simulink model "new_control"  (R2024b)
settings: Solver=FixedStepAuto  StartTime=0.0  StopTime=inf  FixedStep=0.01  RelTol=1e-3  EnableMultiTasking=on
undefined symbols (not defined in the file or in its folder): Discrete, qbreak, Time
libraries: simulink x70, arduinolib x30, dspswit3 x13, arduinosensorlib x2, ctrlSharedLib x2
(part 1 of 4)

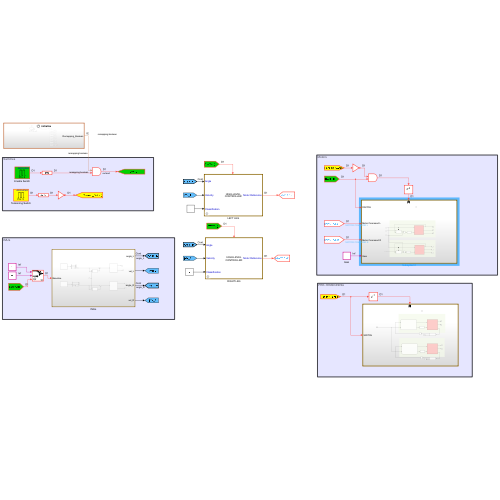
[thumbnail: Simulink's stored preview of the top-level diagram]
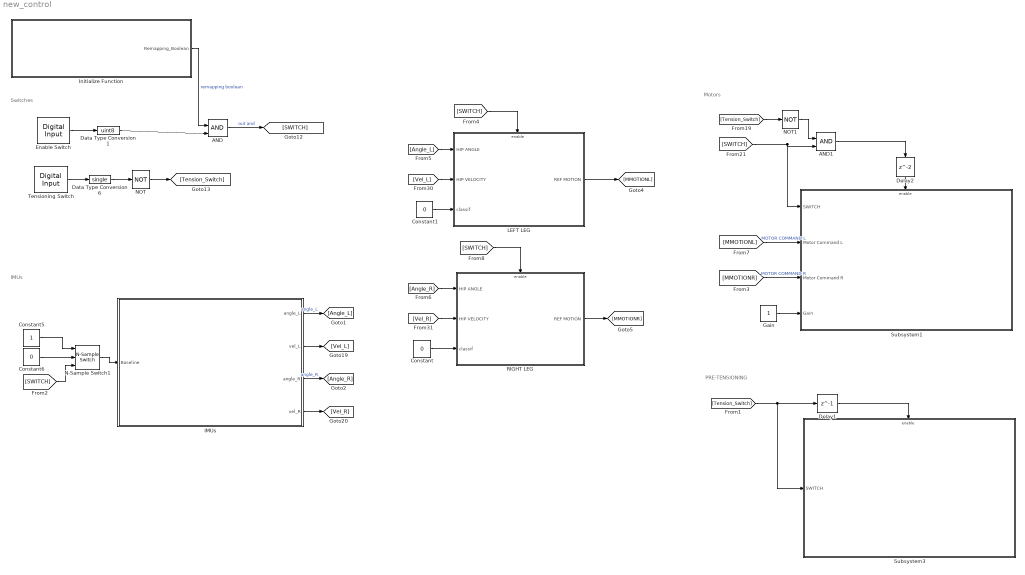
== system new_control ==
  note: Motors
  note: PRE-TENSIONING
  note: IMUs
  note: Switches
  AND : Logic  IconShape=distinctive  AllPortsSameDT=off  OutDataTypeStr=boolean
  AND1 : Logic  IconShape=distinctive  AllPortsSameDT=off  OutDataTypeStr=boolean
  Constant : Constant  Value=0
  Constant1 : Constant  Value=0
  Constant5 : Constant
  Constant6 : Constant  Value=0
  Data Type Conversion1 : DataTypeConversion  OutDataTypeStr=uint8  SaturateOnIntegerOverflow=off  RndMeth=Floor
  Data Type Conversion6 : DataTypeConversion  OutDataTypeStr=single  SaturateOnIntegerOverflow=off  RndMeth=Floor
  Delay1 : Delay  DelayLength=1
  Delay2 : Delay
  Enable Switch : arduinolib/Digital Input  pinNumber=6  mode=Default  Direction=input  SampleTime=0.01  blockPlatform=arduino
  Gain : Constant
  IMUs : Subsystem
  Initialize Function : Subsystem  TreatAsAtomicUnit=on
  LEFT LEG : Subsystem  mask{AMPL=-6.5, LAG=0, SIG_POWER=50}
      mask prompts: AMPL "Motor position desidered amplitude (rad)"; LAG "Lag compensation (rad)"; SIG_POWER "Sigmoid Power"
  N-Sample Switch1 : dspswit3/N-Sample Switch  N=10  reset=on  TriggerType=Rising edge  Ts=0.01
  NOT : Logic  Operator=NOT  IconShape=distinctive  AllPortsSameDT=off  OutDataTypeStr=boolean
  NOT1 : Logic  Operator=NOT  IconShape=distinctive  AllPortsSameDT=off  OutDataTypeStr=boolean
  RIGHT LEG : Subsystem  mask{AMPL=6.5, LAG=0, SIG_POWER=50}
      mask prompts: AMPL "Motor position desidered amplitude (rad)"; LAG "Lag compensation (rad)"; SIG_POWER "Sigmoid Power"
  Subsystem1 : Subsystem
  Subsystem3 : Subsystem
  Tensioning Switch : arduinolib/Digital Input  pinNumber=5  mode=Input Pullup  Direction=input  SampleTime=0.01  blockPlatform=arduino
  wires:
  LEFT LEG/1(REF MOTION) -> [MMOTIONL]
  Gain/1 -> Subsystem1/4(Gain)
  Delay2/1 -> Subsystem1/Enable
  NOT1/1 -> AND1/1
  AND1/1 -> Delay2/1
  [SWITCH] -> AND1/2, Subsystem1/1(SWITCH)
  [Tension_Switch] -> NOT1/1
  Delay1/1 -> Subsystem3/Enable
  [Tension_Switch] -> Subsystem3/1(SWITCH), Delay1/1
  IMUs/1(angle_L) -> [Angle_L]  "angle_L"
  N-Sample Switch1/1 -> IMUs/1(Baseline)
  Constant6/1 -> N-Sample Switch1/2
  Constant5/1 -> N-Sample Switch1/1
  IMUs/3(angle_R) -> [Angle_R]  "angle_R"
  [SWITCH] -> N-Sample Switch1/3
  [SWITCH] -> LEFT LEG/Enable
  [Angle_L] -> LEFT LEG/1(HIP ANGLE)
  Tensioning Switch/1 -> Data Type Conversion6/1
  Data Type Conversion1/1 -> AND/2
  NOT/1 -> [Tension_Switch]
  Initialize Function/1(Remapping_Boolean) -> AND/1  "remapping boolean"
  Data Type Conversion6/1 -> NOT/1
  AND/1 -> [SWITCH]  "out and"
  Enable Switch/1 -> Data Type Conversion1/1
  [Angle_R] -> RIGHT LEG/1(HIP ANGLE)
  [MMOTIONL] -> Subsystem1/2(Motor Command L)  "MOTOR COMMAND L"
  [MMOTIONR] -> Subsystem1/3(Motor Command R)  "MOTOR COMMAND R"
  RIGHT LEG/1(REF MOTION) -> [MMOTIONR]
  [SWITCH] -> RIGHT LEG/Enable
  Constant1/1 -> LEFT LEG/3(classif)
  Constant/1 -> RIGHT LEG/3(classif)
  IMUs/2(vel_L) -> [Vel_L]
  IMUs/4(vel_R) -> [Vel_R]
  [Vel_L] -> LEFT LEG/2(HIP VELOCITY)
  [Vel_R] -> RIGHT LEG/2(HIP VELOCITY)

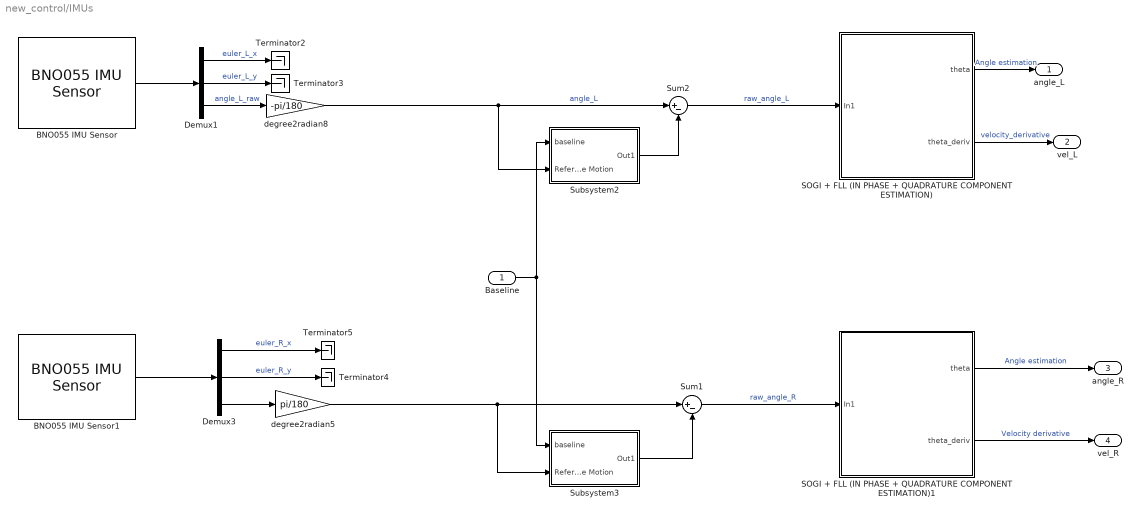
== system new_control/IMUs ==
  Baseline : Inport
  BNO055 IMU Sensor : arduinosensorlib/BNO055 IMU Sensor  I2CModule=0  SlaveAddress=0x28  OperationMode=Fusion  Accel=off  AngularRate=off  MagField=off  EulerAngles=on  Quat=off  LinearAccel=off  GravityVector=off  Status=off  Timestamp=off  AccelRange=4G  AccelBW=62.5 Hz  GyroRange=2000 dps  GyroBW=32 Hz  MagODR=10 Hz  spf=1  SampleTime=-1  blockPlatform=ARDUINO  QueueSizeFactor=1
  BNO055 IMU Sensor1 : arduinosensorlib/BNO055 IMU Sensor  I2CModule=0  SlaveAddress=0x29  OperationMode=Fusion  Accel=off  AngularRate=off  MagField=off  EulerAngles=on  Quat=off  LinearAccel=off  GravityVector=off  Status=off  Timestamp=off  AccelRange=4G  AccelBW=62.5 Hz  GyroRange=2000 dps  GyroBW=32 Hz  MagODR=10 Hz  spf=1  SampleTime=-1  blockPlatform=ARDUINO  QueueSizeFactor=1
  Demux1 : Demux  Outputs=3
  Demux3 : Demux  Outputs=3
  SOGI + FLL (IN PHASE + QUADRATURE COMPONENT ESTIMATION) : Subsystem  mask{Tsamp=0.01, fmin=0.2, fmax=4.0, ksogi=1, kfll=1.0, Elo=1e-4, Ehi=1e-2}
      mask prompts: Tsamp "Sampling time (s)"; fmin "Minimum movement frequency (Hz)"; fmax "Maximum movement frequency (Hz)"; ksogi "SOGI amplitude adaptation gain"; kfll "FLL frequency adaptation gain"; Elo "Low energy threshold"; Ehi "High energy threshold"
  SOGI + FLL (IN PHASE + QUADRATURE COMPONENT ESTIMATION)1 : Subsystem  mask{Tsamp=0.01, fmin=0.2, fmax=4.0, ksogi=1, kfll=1.0, Elo=1e-4, Ehi=1e-2}
      mask prompts: Tsamp "Sampling time (s)"; fmin "Minimum movement frequency (Hz)"; fmax "Maximum movement frequency (Hz)"; ksogi "SOGI amplitude adaptation gain"; kfll "FLL frequency adaptation gain"; Elo "Low energy threshold"; Ehi "High energy threshold"
  Subsystem2 : Subsystem
  Subsystem3 : Subsystem
  Sum1 : Sum  Inputs=|+-
  Sum2 : Sum  Inputs=|+-
  Terminator{2..5} (4 alike) : Terminator
  degree2radian5 : Gain  Gain=pi/180
  degree2radian8 : Gain  Gain=-pi/180
  angle_L : Outport
  vel_L : Outport  Port=2
  angle_R : Outport  Port=3
  vel_R : Outport  Port=4
  wires:
  BNO055 IMU Sensor/1 -> Demux1/1
  BNO055 IMU Sensor1/1 -> Demux3/1
  Demux1/1 -> Terminator2/1  "euler_L_x"
  Demux1/3 -> degree2radian8/1  "angle_L_raw"
  Demux1/2 -> Terminator3/1  "euler_L_y"
  Demux3/1 -> Terminator5/1  "euler_R_x"
  Demux3/2 -> Terminator4/1  "euler_R_y"
  Demux3/3 -> degree2radian5/1
  Sum1/1 -> SOGI + FLL (IN PHASE + QUADRATURE COMPONENT ESTIMATION)1/1(In1)  "raw_angle_R"
  Baseline/1 -> Subsystem2/1(baseline), Subsystem3/1(baseline)
  Subsystem2/1(Out1) -> Sum2/2
  degree2radian5/1 -> Subsystem3/2(Reference Motion), Sum1/1
  Subsystem3/1(Out1) -> Sum1/2
  degree2radian8/1 -> Subsystem2/2(Reference Motion), Sum2/1  "angle_L"
  Sum2/1 -> SOGI + FLL (IN PHASE + QUADRATURE COMPONENT ESTIMATION)/1(In1)  "raw_angle_L"
  SOGI + FLL (IN PHASE + QUADRATURE COMPONENT ESTIMATION)/1(theta) -> angle_L/1  "Angle estimation"
  SOGI + FLL (IN PHASE + QUADRATURE COMPONENT ESTIMATION)1/1(theta) -> angle_R/1  "Angle estimation"
  SOGI + FLL (IN PHASE + QUADRATURE COMPONENT ESTIMATION)1/2(theta_deriv) -> vel_R/1  "Velocity derivative"
  SOGI + FLL (IN PHASE + QUADRATURE COMPONENT ESTIMATION)/2(theta_deriv) -> vel_L/1  "velocity_derivative"

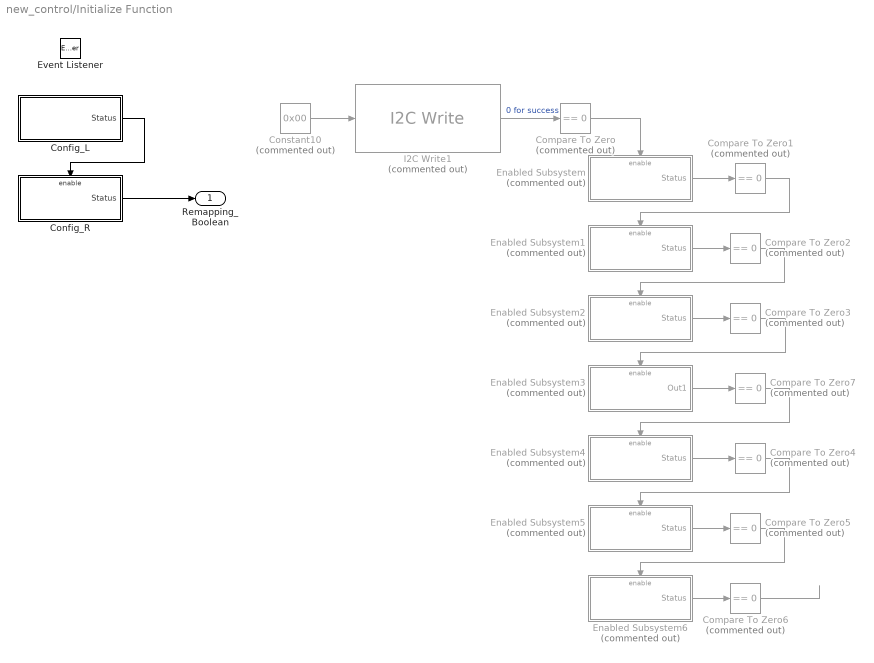
== system new_control/Initialize Function ==
  Compare To Zero{,1..7} (8 alike) : simulink/Logic and Bit Operations/Compare To Zero  Commented=on  relop===  OutDataTypeStr=boolean
  "Config_L " : Subsystem  TreatAsAtomicUnit=on
  Config_R : Subsystem  TreatAsAtomicUnit=on
  Constant10 : Constant  Commented=on  Value=0x00
  Enabled Subsystem : Subsystem  Commented=on  TreatAsAtomicUnit=on
  Enabled Subsystem1 : Subsystem  Commented=on  TreatAsAtomicUnit=on
  Enabled Subsystem2 : Subsystem  Commented=on  TreatAsAtomicUnit=on
  Enabled Subsystem3 : Subsystem  Commented=on  TreatAsAtomicUnit=on
  Enabled Subsystem4 : Subsystem  Commented=on  TreatAsAtomicUnit=on
  Enabled Subsystem5 : Subsystem  Commented=on  TreatAsAtomicUnit=on
  Enabled Subsystem6 : Subsystem  Commented=on  TreatAsAtomicUnit=on
  Event Listener : EventListener  DisableCoverage=on  EventName=reset
  I2C Write1 : arduinolib/I2C Write  Commented=on  I2CModule=0  Mode=Master  SlaveAddress=0x29  SlaveByteOrder=BigEndian  Direction=Transmitter  RegisterAddressMode=on  RegisterAddress=0x3D  SlaveDataType=uint8  DataLength=1  NoAck=off  RepeatedStart=off  OutputStatus=on  blockPlatform=ARDUINO
  Remapping_Boolean : Outport
  wires:
  Compare To Zero/1 -> Enabled Subsystem/Enable
  I2C Write1/1 -> Compare To Zero/1  "0 for success"
  Constant10/1 -> I2C Write1/1
  Enabled Subsystem/1(Status) -> Compare To Zero1/1
  Compare To Zero1/1 -> Enabled Subsystem1/Enable
  Enabled Subsystem1/1(Status) -> Compare To Zero2/1
  Compare To Zero2/1 -> Enabled Subsystem2/Enable
  Enabled Subsystem2/1(Status) -> Compare To Zero3/1
  Compare To Zero3/1 -> Enabled Subsystem3/Enable
  Enabled Subsystem5/1(Status) -> Compare To Zero5/1
  Enabled Subsystem6/1(Status) -> Compare To Zero6/1
  Compare To Zero4/1 -> Enabled Subsystem5/Enable
  Enabled Subsystem4/1(Status) -> Compare To Zero4/1
  Compare To Zero5/1 -> Enabled Subsystem6/Enable
  Enabled Subsystem3/1(Out1) -> Compare To Zero7/1
  Compare To Zero7/1 -> Enabled Subsystem4/Enable
  Compare To Zero6/1 -> ?
  "Config_L "/1(Status) -> Config_R/Enable
  Config_R/1(Status) -> Remapping_Boolean/1

== system new_control/LEFT LEG ==
  note: AMPLITUDE MODULATION
  note: GAIT PHASE
  HIP ANGLE : Inport
  HIP VELOCITY : Inport  Port=2
  classif : Inport  Port=3
  Enable : EnablePort  StatesWhenEnabling=reset
  GAIT PHASE BLOCK : Subsystem
  Lag compensation : Constant  Value=LAG
  MOTOR POSITION REFERENCE GENERATOR : Subsystem
  Reference amplitude : Constant  Value=AMPL
  Sigmoid Power : Constant  Value=SIG_POWER
  Subsystem : Subsystem
  REF MOTION : Outport
  wires:
  Lag compensation/1 -> MOTOR POSITION REFERENCE GENERATOR/2(LAG COMPENSATION)
  GAIT PHASE BLOCK/1(GAIT PHASE) -> MOTOR POSITION REFERENCE GENERATOR/1(GAIT PHASE)
  HIP ANGLE/1 -> GAIT PHASE BLOCK/1(angle), Subsystem/1(Angle estimation)
  Subsystem/1(Out1) -> MOTOR POSITION REFERENCE GENERATOR/3(AMPLITUDE)
  MOTOR POSITION REFERENCE GENERATOR/1(Ref motion) -> REF MOTION/1  "Motor Command"
  HIP VELOCITY/1 -> Subsystem/2(Velocity surrogate (quarature component)), GAIT PHASE BLOCK/2(velocity)
  classif/1 -> Subsystem/3(classif)
  Reference amplitude/1 -> Subsystem/4(Ref amplitude)
  Sigmoid Power/1 -> Subsystem/5(sig_power)

== system new_control/RIGHT LEG ==
  note: AMPLITUDE MODULATION
  note: GAIT PHASE
  HIP ANGLE : Inport
  HIP VELOCITY : Inport  Port=2
  classif : Inport  Port=3
  Enable : EnablePort  StatesWhenEnabling=reset
  GAIT PHASE BLOCK : Subsystem
  Lag compensation : Constant  Value=LAG
  MOTOR POSITION REFERENCE GENERATOR : Subsystem
  Reference amplitude : Constant  Value=AMPL
  Sigmoid Power : Constant  Value=SIG_POWER
  Subsystem : Subsystem
  REF MOTION : Outport
  wires:
  Lag compensation/1 -> MOTOR POSITION REFERENCE GENERATOR/2(LAG COMPENSATION)
  GAIT PHASE BLOCK/1(GAIT PHASE) -> MOTOR POSITION REFERENCE GENERATOR/1(GAIT PHASE)
  HIP VELOCITY/1 -> GAIT PHASE BLOCK/2(velocity), Subsystem/2(Velocity surrogate (quarature component))
  HIP ANGLE/1 -> GAIT PHASE BLOCK/1(angle), Subsystem/1(Angle estimation)
  Subsystem/1(Amplitude_R) -> MOTOR POSITION REFERENCE GENERATOR/3(AMPLITUDE)
  MOTOR POSITION REFERENCE GENERATOR/1(Ref motion) -> REF MOTION/1
  Reference amplitude/1 -> Subsystem/3(Ref amplitude)
  classif/1 -> Subsystem/4(classif)
  Sigmoid Power/1 -> Subsystem/5(Sig_Power)

== system new_control/Subsystem1 ==
  note: LeftLeg_AK60-6 Motor Modules
  note: RightLeg_AK60-6 Motor Modules
  SWITCH : Inport
  Motor Command L : Inport  Port=2
  Motor Command R : Inport  Port=3
  Gain : Inport  Port=4
  Enable : EnablePort  StatesWhenEnabling=reset
  Data Type Conversion1 : DataTypeConversion  OutDataTypeStr=single  SaturateOnIntegerOverflow=off  RndMeth=Floor
  Data Type Conversion2 : DataTypeConversion  OutDataTypeStr=single  SaturateOnIntegerOverflow=off  RndMeth=Floor
  Left Motor Velocity1 : Subsystem
  PID1 : Subsystem
  PID2 : Subsystem
  Product : Product
  Product1 : Product
  Right Motor Velocity1 : Subsystem
  Terminator{,1..5} (6 alike) : Terminator
  wires:
  Motor Command L/1 -> PID1/1(Ref)
  PID1/1(Velocity output) -> Product/1
  Left Motor Velocity1/1(MOTOR POSITION) -> Terminator3/1, PID1/2(Actual Motion)  "Motor_Position_L"
  Data Type Conversion1/1 -> Left Motor Velocity1/2(Motor command)
  Motor Command R/1 -> PID2/1(Ref)
  PID2/1(Velocity output) -> Product1/2
  SWITCH/1 -> Right Motor Velocity1/1(SWITCH), PID2/Enable, PID1/Enable, Left Motor Velocity1/1(SWITCH)
  Data Type Conversion2/1 -> Right Motor Velocity1/2(Motor command)
  Left Motor Velocity1/3(MOTOR TORQUE) -> Terminator5/1  "Motor_Torque_L"
  Left Motor Velocity1/2(MOTOR SPEED) -> Terminator4/1  "Motor_Speed_L"
  Right Motor Velocity1/1(MOTOR POSITION) -> Terminator/1, PID2/2(Actual Motion)  "Motor_Position_R"
  Right Motor Velocity1/2(MOTOR SPEED) -> Terminator1/1  "Motor_Speed_R"
  Right Motor Velocity1/3(MOTOR TORQUE) -> Terminator2/1  "Motor_Torque_R"
  Product/1 -> Data Type Conversion1/1
  Product1/1 -> Data Type Conversion2/1
  Gain/1 -> Product1/1, Product/2

== system new_control/Subsystem3 ==
  note: RightLeg_AK60-6 Motor Modules
  note: LeftLeg_AK60-6 Motor Modules
  SWITCH : Inport
  Enable : EnablePort  StatesWhenEnabling=reset
  Abs : Abs  SaturateOnIntegerOverflow=off
  Abs1 : Abs  SaturateOnIntegerOverflow=off
  Chart : Stateflow chart  TreatAsAtomicUnit=on
  Chart1 : Stateflow chart  TreatAsAtomicUnit=on
  Data Type Conversion1 : DataTypeConversion  OutDataTypeStr=single  SaturateOnIntegerOverflow=off  RndMeth=Floor
  Data Type Conversion6 : DataTypeConversion  OutDataTypeStr=single  SaturateOnIntegerOverflow=off  RndMeth=Floor
  Left Motor Velocity : Subsystem
  Right Motor Velocity : Subsystem
  Subsystem1 : Subsystem  mask{wn=25, zt=1, x0=0}
      mask prompts: wn "Cut-off frequency (rad/s)"; zt "Damping ratio"; x0 "Initial Condition"
  Subsystem4 : Subsystem  mask{wn=25, zt=1, x0=0}
      mask prompts: wn "Cut-off frequency (rad/s)"; zt "Damping ratio"; x0 "Initial Condition"
  Terminator{1..6} (6 alike) : Terminator
  wires:
  Chart1/2(vel) -> Data Type Conversion1/1
  SWITCH/1 -> Chart1/2(ON_OFF), Chart/2(ON_OFF)
  Data Type Conversion6/1 -> Right Motor Velocity/2(Motor command)
  Left Motor Velocity/3(MOTOR TORQUE) -> Subsystem1/1(x)
  Right Motor Velocity/2(MOTOR SPEED) -> Terminator2/1
  Left Motor Velocity/2(MOTOR SPEED) -> Terminator1/1
  Chart/2(vel) -> Data Type Conversion6/1
  Right Motor Velocity/1(MOTOR POSITION) -> Terminator4/1
  Subsystem4/1(y) -> Abs/1  "TORQUE"
  Right Motor Velocity/3(MOTOR TORQUE) -> Subsystem4/1(x)
  Subsystem4/2(yd) -> Terminator5/1
  Abs/1 -> Chart/1(MOTOR_TORQUE)
  Left Motor Velocity/1(MOTOR POSITION) -> Terminator3/1
  Subsystem1/1(y) -> Abs1/1  "TORQUE"
  Subsystem1/2(yd) -> Terminator6/1
  Abs1/1 -> Chart1/1(MOTOR_TORQUE)
  Chart/1(enablestati) -> Right Motor Velocity/1(SWITCH)
  Chart1/1(enablestati) -> Left Motor Velocity/1(SWITCH)
  Data Type Conversion1/1 -> Left Motor Velocity/2(Motor command)

== system new_control/IMUs/SOGI + FLL (IN PHASE + QUADRATURE COMPONENT ESTIMATION) ==
  note: %% ---- TUNING----%%
      |
      | f_min % Minimum expected cadence (Hz): lower if very slow walking is possible
      | f_max % Maximum expected cadence (Hz): increase if including fast walking/running
      |
      | k_sogi % Tune k_sogi only if the portrait is ringy or too sluggish:
      | % Increase to 1.2–1.4 if theta/theta_quad look underdamped / not tracking well
      | % Decrease to 0.8–0.9 if very noisy and you see jitter
      |
      | k_fll % Frequency adaptation speed: increase to track speed changes faster, decrease if noisy/jittery
      |
      | E_lo % Energy threshold to block adaptation during noise/standing: increase if false locking occurs
      | E_hi % Energy threshold for full adaptation: decrease if it never locks during slow gait
      |
      | OTHER PARAMETERS TO BE TUNED INSIDE THE MATLAB FUNCTION (for walking/running there should not be the need)
  In1 : Inport
  Constant1 : Constant  Value=Tsamp
  Constant2 : Constant  Value=ksogi
  Constant3 : Constant  Value=fmin
  Constant4 : Constant  Value=fmax
  Constant5 : Constant  Value=kfll
  Constant6 : Constant  Value=Ehi
  Constant7 : Constant  Value=Elo
  Discrete Derivative : simulink/Discrete/Discrete Derivative  gainval=1.0  ICPrevScaledInput=0.0  OutMin=[]  OutMax=[]  OutDataType=fixdt(1, 16)  OutScaling=2^-10  DoSatur=off
  MATLAB Function1 : MATLAB Function  TreatAsAtomicUnit=on
  Minus : Sum  Inputs=+-
  REMOVE DRIFT : Subsystem  mask{wn=1.25, zt=1, x0=0}
      mask prompts: wn "Cut-off frequency (rad/s)"; zt "Damping ratio"; x0 "Initial Condition"
  theta_quad : Terminator
  theta : Outport
  theta_deriv : Outport  Port=2
  wires:
  Minus/1 -> MATLAB Function1/1(x)
  Constant3/1 -> MATLAB Function1/3(f_min)
  Constant4/1 -> MATLAB Function1/4(f_max)
  REMOVE DRIFT/1(y) -> Minus/2
  Constant5/1 -> MATLAB Function1/6(k_fll)
  Constant6/1 -> MATLAB Function1/8(E_hi)
  Constant1/1 -> MATLAB Function1/2(Ts)
  Constant7/1 -> MATLAB Function1/7(E_lo)
  In1/1 -> REMOVE DRIFT/1(x), Minus/1
  Constant2/1 -> MATLAB Function1/5(k_sogi)
  MATLAB Function1/1(theta) -> Discrete Derivative/1, theta/1
  Discrete Derivative/1 -> theta_deriv/1
  MATLAB Function1/2(theta_quad) -> theta_quad/1  "Velocity surrogate  (quarature component)"

== system new_control/IMUs/SOGI + FLL (IN PHASE + QUADRATURE COMPONENT ESTIMATION)1 ==
  note: %% ---- TUNING----%%
      |
      | f_min % Minimum expected cadence (Hz): lower if very slow walking is possible
      | f_max % Maximum expected cadence (Hz): increase if including fast walking/running
      |
      | k_sogi % Tune k_sogi only if the portrait is ringy or too sluggish:
      | % Increase to 1.2–1.4 if theta/theta_quad look underdamped / not tracking well
      | % Decrease to 0.8–0.9 if very noisy and you see jitter
      |
      | k_fll % Frequency adaptation speed: increase to track speed changes faster, decrease if noisy/jittery
      |
      | E_lo % Energy threshold to block adaptation during noise/standing: increase if false locking occurs
      | E_hi % Energy threshold for full adaptation: decrease if it never locks during slow gait
      |
      | OTHER PARAMETERS TO BE TUNED INSIDE THE MATLAB FUNCTION (for walking/running there should not be the need)
  In1 : Inport
  Constant1 : Constant  Value=Tsamp
  Constant2 : Constant  Value=ksogi
  Constant3 : Constant  Value=fmin
  Constant4 : Constant  Value=fmax
  Constant5 : Constant  Value=kfll
  Constant6 : Constant  Value=Ehi
  Constant7 : Constant  Value=Elo
  Discrete Derivative : simulink/Discrete/Discrete Derivative  gainval=1.0  ICPrevScaledInput=0.0  OutMin=[]  OutMax=[]  OutDataType=fixdt(1, 16)  OutScaling=2^-10  DoSatur=off
  MATLAB Function1 : MATLAB Function  TreatAsAtomicUnit=on
  Minus : Sum  Inputs=+-
  REMOVE DRIFT : Subsystem  mask{wn=1.25, zt=1, x0=0}
      mask prompts: wn "Cut-off frequency (rad/s)"; zt "Damping ratio"; x0 "Initial Condition"
  theta_quad : Terminator
  theta : Outport
  theta_deriv : Outport  Port=2
  wires:
  Minus/1 -> MATLAB Function1/1(x)
  Constant3/1 -> MATLAB Function1/3(f_min)
  Constant4/1 -> MATLAB Function1/4(f_max)
  REMOVE DRIFT/1(y) -> Minus/2
  Constant5/1 -> MATLAB Function1/6(k_fll)
  Constant6/1 -> MATLAB Function1/8(E_hi)
  Constant1/1 -> MATLAB Function1/2(Ts)
  Constant7/1 -> MATLAB Function1/7(E_lo)
  In1/1 -> REMOVE DRIFT/1(x), Minus/1
  Constant2/1 -> MATLAB Function1/5(k_sogi)
  MATLAB Function1/1(theta) -> Discrete Derivative/1, theta/1
  Discrete Derivative/1 -> theta_deriv/1
  MATLAB Function1/2(theta_quad) -> theta_quad/1  "Velocity surrogate  (quarature component)"

== system new_control/IMUs/Subsystem2 ==
  baseline : Inport
  Reference Motion : Inport  Port=2
  Delay : Delay
  Memory1 : Memory
  Switch1 : Switch  Criteria=u2 > Threshold  SaturateOnIntegerOverflow=off  InputSameDT=off
  Out1 : Outport
  wires:
  Switch1/1 -> Delay/1, Out1/1
  Memory1/1 -> Switch1/3
  baseline/1 -> Switch1/2
  Reference Motion/1 -> Switch1/1
  Delay/1 -> Memory1/1

== system new_control/IMUs/Subsystem3 ==
  baseline : Inport
  Reference Motion : Inport  Port=2
  Delay : Delay
  Memory1 : Memory
  Switch1 : Switch  Criteria=u2 > Threshold  SaturateOnIntegerOverflow=off  InputSameDT=off
  Out1 : Outport
  wires:
  Switch1/1 -> Delay/1, Out1/1
  Memory1/1 -> Switch1/3
  baseline/1 -> Switch1/2
  Reference Motion/1 -> Switch1/1
  Delay/1 -> Memory1/1

== system new_control/Initialize Function/Config_L  ==
  Enter Config Mode : Subsystem
  Start Fused (NDOF) Mode : Subsystem  TreatAsAtomicUnit=on
  "X=Z, Y=Y, Z=X" : Subsystem
  Z = -Z : Subsystem  TreatAsAtomicUnit=on
  Status : Outport
  wires:
  Enter Config Mode/1(Status) -> "X=Z, Y=Y, Z=X"/Enable
  Z = -Z/1(Status) -> Start Fused (NDOF) Mode/Enable
  Start Fused (NDOF) Mode/1(Status) -> Status/1
  "X=Z, Y=Y, Z=X"/1(Status) -> Z = -Z/Enable

== system new_control/Initialize Function/Config_R ==
  Enable : EnablePort
  Enter Config Mode : Subsystem
  Start Fused (NDOF) Mode : Subsystem  TreatAsAtomicUnit=on
  "X=Z, Y=Y, Z=X" : Subsystem
  Z = -Z : Subsystem  TreatAsAtomicUnit=on
  Status : Outport
  wires:
  Start Fused (NDOF) Mode/1(Status) -> Status/1
  "X=Z, Y=Y, Z=X"/1(Status) -> Z = -Z/Enable
  Z = -Z/1(Status) -> Start Fused (NDOF) Mode/Enable
  Enter Config Mode/1(Status) -> "X=Z, Y=Y, Z=X"/Enable

== system new_control/Initialize Function/Enabled Subsystem ==
  Enable : EnablePort
  Constant13 : Constant  Value=0x06
  I2C Write2 : arduinolib/I2C Write  I2CModule=0  Mode=Master  SlaveAddress=0x29  SlaveByteOrder=BigEndian  Direction=Transmitter  RegisterAddressMode=on  RegisterAddress=0x41  SlaveDataType=uint8  DataLength=1  NoAck=off  RepeatedStart=off  OutputStatus=on  blockPlatform=ARDUINO
  Status : Outport
  wires:
  I2C Write2/1 -> Status/1
  Constant13/1 -> I2C Write2/1

== system new_control/Initialize Function/Enabled Subsystem1 ==
  Enable : EnablePort
  Constant14 : Constant  Value=0x01
  I2C Write3 : arduinolib/I2C Write  I2CModule=0  Mode=Master  SlaveAddress=0x29  SlaveByteOrder=BigEndian  Direction=Transmitter  RegisterAddressMode=on  RegisterAddress=0x42  SlaveDataType=uint8  DataLength=1  NoAck=off  RepeatedStart=off  OutputStatus=on  blockPlatform=ARDUINO
  Status : Outport
  wires:
  I2C Write3/1 -> Status/1
  Constant14/1 -> I2C Write3/1

== system new_control/Initialize Function/Enabled Subsystem2 ==
  Enable : EnablePort
  Constant16 : Constant  Value=0x0C
  I2C Write4 : arduinolib/I2C Write  I2CModule=0  Mode=Master  SlaveAddress=0x29  SlaveByteOrder=BigEndian  Direction=Transmitter  RegisterAddressMode=on  RegisterAddress=0x3D  SlaveDataType=uint8  DataLength=1  NoAck=off  RepeatedStart=off  OutputStatus=on  blockPlatform=ARDUINO
  Status : Outport
  wires:
  Constant16/1 -> I2C Write4/1
  I2C Write4/1 -> Status/1

== system new_control/Initialize Function/Enabled Subsystem3 ==
  Enable : EnablePort
  Constant10 : Constant  Value=0x00
  I2C Write1 : arduinolib/I2C Write  I2CModule=0  Mode=Master  SlaveAddress=0x28  SlaveByteOrder=BigEndian  Direction=Transmitter  RegisterAddressMode=on  RegisterAddress=0x3D  SlaveDataType=uint8  DataLength=1  NoAck=off  RepeatedStart=off  OutputStatus=on  blockPlatform=ARDUINO
  Out1 : Outport
  wires:
  I2C Write1/1 -> Out1/1
  Constant10/1 -> I2C Write1/1

== system new_control/Initialize Function/Enabled Subsystem4 ==
  Enable : EnablePort
  Constant13 : Constant  Value=0x06
  I2C Write2 : arduinolib/I2C Write  I2CModule=0  Mode=Master  SlaveAddress=0x28  SlaveByteOrder=BigEndian  Direction=Transmitter  RegisterAddressMode=on  RegisterAddress=0x41  SlaveDataType=uint8  DataLength=1  NoAck=off  RepeatedStart=off  OutputStatus=on  blockPlatform=ARDUINO
  Status : Outport
  wires:
  I2C Write2/1 -> Status/1
  Constant13/1 -> I2C Write2/1

== system new_control/Initialize Function/Enabled Subsystem5 ==
  Enable : EnablePort
  Constant14 : Constant  Value=0x01
  I2C Write3 : arduinolib/I2C Write  I2CModule=0  Mode=Master  SlaveAddress=0x28  SlaveByteOrder=BigEndian  Direction=Transmitter  RegisterAddressMode=on  RegisterAddress=0x42  SlaveDataType=uint8  DataLength=1  NoAck=off  RepeatedStart=off  OutputStatus=on  blockPlatform=ARDUINO
  Status : Outport
  wires:
  I2C Write3/1 -> Status/1
  Constant14/1 -> I2C Write3/1

== system new_control/Initialize Function/Enabled Subsystem6 ==
  Enable : EnablePort
  Constant16 : Constant  Value=0x0C
  I2C Write4 : arduinolib/I2C Write  I2CModule=0  Mode=Master  SlaveAddress=0x28  SlaveByteOrder=BigEndian  Direction=Transmitter  RegisterAddressMode=on  RegisterAddress=0x3D  SlaveDataType=uint8  DataLength=1  NoAck=off  RepeatedStart=off  OutputStatus=on  blockPlatform=ARDUINO
  Status : Outport
  wires:
  Constant16/1 -> I2C Write4/1
  I2C Write4/1 -> Status/1

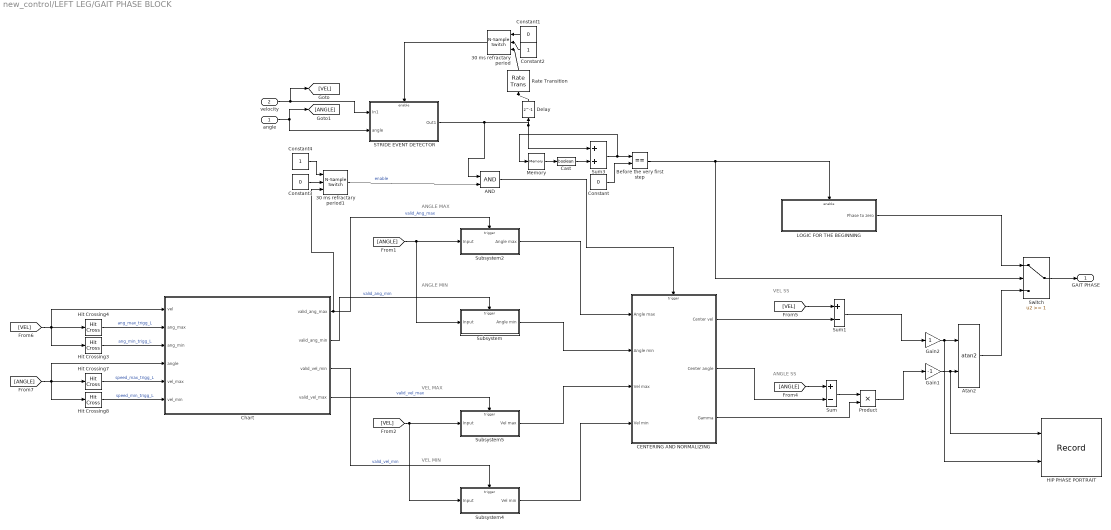
== system new_control/LEFT LEG/GAIT PHASE BLOCK ==
  note: ANGLE MAX
  note: ANGLE MIN
  note: VEL MIN
  note: VEL MAX
  note: ANGLE SS
  note: VEL SS
  angle : Inport
  velocity : Inport  Port=2
  30 ms refractary period : dspswit3/N-Sample Switch  N=30  reset=on  TriggerType=Rising edge  Ts=-1
  30 ms refractary period1 : dspswit3/N-Sample Switch  N=31  reset=on  TriggerType=Rising edge  Ts=0.01
  AND : Logic  IconShape=distinctive  AllPortsSameDT=off  OutDataTypeStr=boolean
  Atan2 : Trigonometry  Operator=atan2  NumberOfIterations=5
  Before the very first step : RelationalOperator  Operator===  OutDataTypeStr=boolean  RndMeth=Simplest  InputSameDT=off
  CENTERING AND NORMALIZING : Subsystem
  Cast : DataTypeConversion  OutDataTypeStr=boolean  SaturateOnIntegerOverflow=off  RndMeth=Floor
  Chart : Stateflow chart  TreatAsAtomicUnit=on
  Constant : Constant  Value=0
  Constant1 : Constant  Value=0
  Constant2 : Constant
  Constant3 : Constant  Value=0
  Constant4 : Constant
  Delay : Delay  DelayLength=1
  Gain1 : Gain  Gain=-1
  Gain2 : Gain
  HIP PHASE PORTRAIT : Record  FileSettingsInternal="{\"entries\":[{\"content\":{\"excelSettings\":{\"content\":{},\"type\":\"Streamout.ExcelSettings\"}},\"type\":\"Streamout.FileSettingStorage\",\"uuid\":\"\"}],\"packageUris\":[\"http:\\/\\/schema.mathworks.com\\/mf0\\/streamout_blocks\\/R2020a\"],\"version\":\"1.0\"}"  Layout=[1 1]  SignalsInternal="{\"entries\":[{\"content\":{},\"type\":\"RecordBlkView.InputSignals\",\"uuid\":\"\"}],\"packageUris\":[\"http:\\/\\/schema.mathworks.com\\/mf0\\/streamout_blocks\\/R2020a\"],\"version\":\"1.0\"}"  VisualizationBindings="{\"xyplotplugin\":{\"info\":[{\"series\":[],\"subplotID\":1}]}}"  CompatibilityTag=XY
  Hit Crossing3 : HitCross  HitCrossingDirection=rising
  Hit Crossing4 : HitCross  HitCrossingDirection=falling
  Hit Crossing7 : HitCross  HitCrossingDirection=rising
  Hit Crossing8 : HitCross  HitCrossingDirection=falling
  LOGIC FOR THE BEGINNING : Subsystem
  Memory : Memory
  Product : Product
  Rate Transition : RateTransition  OutPortSampleTime=0.01
  STRIDE EVENT DETECTOR : Subsystem
  Subsystem : Subsystem
  Subsystem2 : Subsystem
  Subsystem4 : Subsystem
  Subsystem5 : Subsystem
  Sum : Sum  Inputs=+-
  Sum1 : Sum  Inputs=+-
  Sum3 : Sum
  Switch : Switch  Threshold=1  SaturateOnIntegerOverflow=off  InputSameDT=off
  GAIT PHASE : Outport
  wires:
  angle/1 -> [ANGLE], STRIDE EVENT DETECTOR/2(angle)
  velocity/1 -> STRIDE EVENT DETECTOR/1(In1), [VEL]
  [ANGLE] -> Subsystem/1(Input), Subsystem2/1(Input)
  [VEL] -> Subsystem4/1(Input), Subsystem5/1(Input)
  STRIDE EVENT DETECTOR/1(Out1) -> AND/1, Sum3/1, Delay/1
  Subsystem2/1(Angle max) -> CENTERING AND NORMALIZING/1(Angle max)
  Subsystem/1(Angle min) -> CENTERING AND NORMALIZING/2(Angle min)
  Subsystem5/1(Vel max) -> CENTERING AND NORMALIZING/3(Vel max)
  Subsystem4/1(Vel min) -> CENTERING AND NORMALIZING/4(Vel min)
  [ANGLE] -> Sum/1
  CENTERING AND NORMALIZING/2(Center angle) -> Sum/2
  Sum/1 -> Product/1
  CENTERING AND NORMALIZING/3(Gamma) -> Product/2
  Product/1 -> Gain1/1
  [VEL] -> Sum1/1
  CENTERING AND NORMALIZING/1(Center vel) -> Sum1/2
  Sum1/1 -> Gain2/1
  Atan2/1 -> Switch/3
  Gain1/1 -> HIP PHASE PORTRAIT/1, Atan2/2
  Sum3/1 -> Memory/1, Before the very first step/1
  Constant/1 -> Before the very first step/2
  Before the very first step/1 -> Switch/2, LOGIC FOR THE BEGINNING/Enable
  LOGIC FOR THE BEGINNING/1(Phase to zero) -> Switch/1
  Switch/1 -> GAIT PHASE/1
  Memory/1 -> Cast/1
  Cast/1 -> Sum3/2
  30 ms refractary period/1 -> STRIDE EVENT DETECTOR/Enable
  Constant1/1 -> 30 ms refractary period/1
  Constant2/1 -> 30 ms refractary period/2
  Delay/1 -> Rate Transition/1
  Gain2/1 -> HIP PHASE PORTRAIT/2, Atan2/1
  Rate Transition/1 -> 30 ms refractary period/3
  [VEL] -> Chart/5(vel), Hit Crossing3/1, Hit Crossing4/1
  Hit Crossing3/1 -> Chart/4(ang_min)  "ang_min_trigg_L"
  Hit Crossing4/1 -> Chart/1(ang_max)  "ang_max_trigg_L"
  [ANGLE] -> Chart/6(angle), Hit Crossing8/1, Hit Crossing7/1
  Hit Crossing7/1 -> Chart/3(vel_max)  "speed_max_trigg_L"
  Hit Crossing8/1 -> Chart/2(vel_min)  "speed_min_trigg_L"
  Chart/4(valid_ang_min) -> Subsystem/Trigger  "valid_ang_min"
  Chart/2(valid_vel_min) -> Subsystem4/Trigger  "valid_vel_min"
  Chart/1(valid_vel_max) -> Subsystem5/Trigger  "valid_vel_max"
  Chart/3(valid_ang_max) -> 30 ms refractary period1/3, Subsystem2/Trigger  "valid_Ang_max"
  Constant3/1 -> 30 ms refractary period1/2
  30 ms refractary period1/1 -> AND/2  "enable"
  Constant4/1 -> 30 ms refractary period1/1
  AND/1 -> CENTERING AND NORMALIZING/Trigger

== system new_control/LEFT LEG/MOTOR POSITION REFERENCE GENERATOR ==
  note: KALMAN FILTER
  GAIT PHASE : Inport
  LAG COMPENSATION : Inport  Port=2
  AMPLITUDE : Inport  Port=3
  Gain : Gain  Gain=-1
  Motion mapping2 : Lookup_n-D  NumberOfTableDimensions=1  BreakpointsForDimension1=[-1, -0.8, -0.6, -0.4, -0.2, -0.1, 0, 0.1, 0.2, 0.4, 0.6, 0.8, 1]  BreakpointsForDimension2=qbreak(:,2)  Table=[-1, -0.8, -0.6, -0.4, -0.2, -0.1, 0, 0, 0.005, 0.01, 0.015,0.02,0.025]  InterpMethod=Cubic spline  ExtrapMethod=Cubic spline  InternalRulePriority=Speed  RndMeth=Simplest
  Plus : Sum
  Product : Product
  Rate Transition : RateTransition  OutPortSampleTime=0.01
  Ref traj w/ noise : ctrlSharedLib/Kalman Filter  Commented=on  TimeDomain=Discrete-Time  UseCurrentEstimator=off  ModelSource=Individual A, B, C, D matrices  ModelSourceVariable=ss(0.95,1,1,0,1)  A=[1]  B=1  C=[1]  D=0  NumberOfStates=1  NumberOfInputs=1  NumberOfOutputs=1  InitialEstimateSource=Dialog  X0=[0]  P0=10  UseK=off  UseGH=off  NumberOfProcessNoiseInputs=1  G=1  TimeInvariantG=on  H=0  TimeInvariantH=on  Q=1e-3  TimeInvariantQ=on  R=9e-4  TimeInvariantR=on  N=0  TimeInvariantN=on  AddInputPort=off  AddEnablePort=off  OutputEstimatedY=off  OutputP=off  Ts=-1
  Saturation : Saturate  UpperLimit=600*pi/180  LowerLimit=-600*pi/180
  Sin1 : Trigonometry
  Ref motion : Outport
  wires:
  Motion mapping2/1 -> Product/1  "motion_mapping"
  Product/1 -> Saturation/1
  Sin1/1 -> Gain/1
  Plus/1 -> Sin1/1
  GAIT PHASE/1 -> Plus/1
  LAG COMPENSATION/1 -> Plus/2
  AMPLITUDE/1 -> Product/2
  Gain/1 -> Rate Transition/1
  Saturation/1 -> Ref motion/1
  Rate Transition/1 -> Motion mapping2/1

== system new_control/LEFT LEG/Subsystem ==
  Angle estimation : Inport
  Velocity surrogate (quarature component) : Inport  Port=2
  classif : Inport  Port=3
  Ref amplitude : Inport  Port=4
  sig_power : Inport  Port=5
  Cast To Double : DataTypeConversion  OutDataTypeStr=double  SaturateOnIntegerOverflow=off  RndMeth=Floor
  Chart1 : Stateflow chart  TreatAsAtomicUnit=on
  Constant : Constant
  Product : Product
  Product1 : Product
  SIGMOID SCALING : Subsystem
  Sqrt : Sqrt
  Square : Math  Operator=square
  Square1 : Math  Operator=square
  Sum : Sum
  Out1 : Outport
  wires:
  Square/1 -> Sum/1
  Square1/1 -> Sum/2
  Sum/1 -> Sqrt/1
  Product/1 -> Out1/1
  Sqrt/1 -> Product1/1  "PORTRAIT RADIUS"
  SIGMOID SCALING/1(Out1) -> Product/1
  Cast To Double/1 -> Chart1/1(class)
  classif/1 -> Cast To Double/1
  Chart1/3(sigmoid_power) -> SIGMOID SCALING/2(Sigmoid Power)
  Chart1/2(gain) -> Product/2
  Velocity surrogate (quarature component)/1 -> Square1/1
  sig_power/1 -> Chart1/3(sig_power)
  Ref amplitude/1 -> Chart1/2(amplitude)
  Angle estimation/1 -> Square/1
  Product1/1 -> SIGMOID SCALING/1(PORTRAIT RADIUS)
  Chart1/1(scale) -> Product1/2
  Constant/1 -> Chart1/4(Scale_LM)

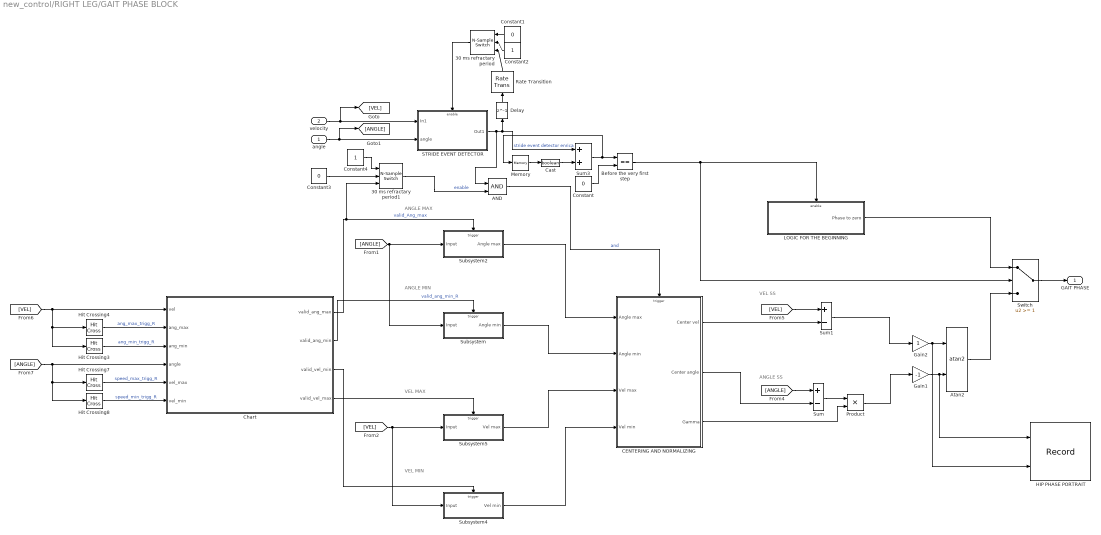
== system new_control/RIGHT LEG/GAIT PHASE BLOCK ==
  note: ANGLE MAX
  note: ANGLE MIN
  note: VEL MIN
  note: VEL MAX
  note: ANGLE SS
  note: VEL SS
  angle : Inport
  velocity : Inport  Port=2
  30 ms refractary period : dspswit3/N-Sample Switch  N=30  reset=on  TriggerType=Rising edge  Ts=-1
  30 ms refractary period1 : dspswit3/N-Sample Switch  N=31  reset=on  TriggerType=Rising edge  Ts=0.01
  AND : Logic  IconShape=distinctive  AllPortsSameDT=off  OutDataTypeStr=boolean
  Atan2 : Trigonometry  Operator=atan2  NumberOfIterations=5
  Before the very first step : RelationalOperator  Operator===  OutDataTypeStr=boolean  RndMeth=Simplest  InputSameDT=off
  CENTERING AND NORMALIZING : Subsystem
  Cast : DataTypeConversion  OutDataTypeStr=boolean  SaturateOnIntegerOverflow=off  RndMeth=Floor
  Chart : Stateflow chart  TreatAsAtomicUnit=on
  Constant : Constant  Value=0
  Constant1 : Constant  Value=0
  Constant2 : Constant
  Constant3 : Constant  Value=0
  Constant4 : Constant
  Delay : Delay  DelayLength=1
  Gain1 : Gain  Gain=-1
  Gain2 : Gain
  HIP PHASE PORTRAIT : Record  FileSettingsInternal="{\"entries\":[{\"content\":{\"excelSettings\":{\"content\":{},\"type\":\"Streamout.ExcelSettings\"}},\"type\":\"Streamout.FileSettingStorage\",\"uuid\":\"\"}],\"packageUris\":[\"http:\\/\\/schema.mathworks.com\\/mf0\\/streamout_blocks\\/R2020a\"],\"version\":\"1.0\"}"  Layout=[1 1]  SignalsInternal="{\"entries\":[{\"content\":{\"signals\":[{\"content\":{\"blockPath\":[],\"dimensions\":[1],\"domain\":\"\",\"lineColor\":\"#ff6929\",\"lineWidth\":2,\"port\":1,\"signalID\":1,\"signalName\":\"Gain1\"},\"type\":\"RecordBlkView.Signal\",\"uuid\":\"\"},{\"content\":{\"blockPath\":[],\"dimensions\":[1],\"domain\":\"\",\"lineColor\":\"#b746ff\",\"lineWidth\":2,\"port\":2,\"signalID\":2,\"signalName\":\"Gain2\"},\"type\":\"RecordBlkView.Signal\",\"uuid\":\"\"}]},\"type\":\"R ...(+134 chars)"  VisualizationBindings="{\"xyplotplugin\":{\"info\":[{\"series\":[],\"subplotID\":1}]}}"  CompatibilityTag=XY
  Hit Crossing3 : HitCross  HitCrossingDirection=rising
  Hit Crossing4 : HitCross  HitCrossingDirection=falling
  Hit Crossing7 : HitCross  HitCrossingDirection=rising
  Hit Crossing8 : HitCross  HitCrossingDirection=falling
  LOGIC FOR THE BEGINNING : Subsystem
  Memory : Memory
  Product : Product
  Rate Transition : RateTransition  OutPortSampleTime=0.01
  STRIDE EVENT DETECTOR : Subsystem
  Subsystem : Subsystem
  Subsystem2 : Subsystem
  Subsystem4 : Subsystem
  Subsystem5 : Subsystem
  Sum : Sum  Inputs=+-
  Sum1 : Sum  Inputs=+-
  Sum3 : Sum
  Switch : Switch  Threshold=1  SaturateOnIntegerOverflow=off  InputSameDT=off
  GAIT PHASE : Outport
  wires:
  angle/1 -> [ANGLE], STRIDE EVENT DETECTOR/2(angle)
  velocity/1 -> STRIDE EVENT DETECTOR/1(In1), [VEL]
  [ANGLE] -> Subsystem/1(Input), Subsystem2/1(Input)
  Chart/2(valid_vel_min) -> Subsystem4/Trigger
  [VEL] -> Subsystem4/1(Input), Subsystem5/1(Input)
  Subsystem2/1(Angle max) -> CENTERING AND NORMALIZING/1(Angle max)
  Subsystem/1(Angle min) -> CENTERING AND NORMALIZING/2(Angle min)
  Subsystem5/1(Vel max) -> CENTERING AND NORMALIZING/3(Vel max)
  Subsystem4/1(Vel min) -> CENTERING AND NORMALIZING/4(Vel min)
  [ANGLE] -> Sum/1
  CENTERING AND NORMALIZING/2(Center angle) -> Sum/2
  Sum/1 -> Product/1
  CENTERING AND NORMALIZING/3(Gamma) -> Product/2
  Product/1 -> Gain1/1
  [VEL] -> Sum1/1
  CENTERING AND NORMALIZING/1(Center vel) -> Sum1/2
  Sum1/1 -> Gain2/1
  Atan2/1 -> Switch/3
  Gain1/1 -> HIP PHASE PORTRAIT/1, Atan2/2
  Sum3/1 -> Memory/1, Before the very first step/1
  Constant/1 -> Before the very first step/2
  Before the very first step/1 -> Switch/2, LOGIC FOR THE BEGINNING/Enable
  LOGIC FOR THE BEGINNING/1(Phase to zero) -> Switch/1
  Switch/1 -> GAIT PHASE/1
  Memory/1 -> Cast/1
  Cast/1 -> Sum3/2
  30 ms refractary period/1 -> STRIDE EVENT DETECTOR/Enable
  Constant1/1 -> 30 ms refractary period/1
  Constant2/1 -> 30 ms refractary period/2
  Delay/1 -> Rate Transition/1
  Gain2/1 -> HIP PHASE PORTRAIT/2, Atan2/1
  Rate Transition/1 -> 30 ms refractary period/3
  Hit Crossing3/1 -> Chart/4(ang_min)  "ang_min_trigg_R"
  [VEL] -> Hit Crossing3/1, Hit Crossing4/1, Chart/5(vel)
  Hit Crossing7/1 -> Chart/3(vel_max)  "speed_max_trigg_R"
  [ANGLE] -> Hit Crossing8/1, Hit Crossing7/1, Chart/6(angle)
  Hit Crossing4/1 -> Chart/1(ang_max)  "ang_max_trigg_R"
  Hit Crossing8/1 -> Chart/2(vel_min)  "speed_min_trigg_R"
  Chart/4(valid_ang_min) -> Subsystem/Trigger  "valid_ang_min_R"
  Chart/1(valid_vel_max) -> Subsystem5/Trigger
  Chart/3(valid_ang_max) -> Subsystem2/Trigger, 30 ms refractary period1/3  "valid_Ang_max"
  Constant3/1 -> 30 ms refractary period1/2
  30 ms refractary period1/1 -> AND/2  "enable"
  STRIDE EVENT DETECTOR/1(Out1) -> AND/1, Delay/1, Sum3/1  "stride event detector enrica"
  Constant4/1 -> 30 ms refractary period1/1
  AND/1 -> CENTERING AND NORMALIZING/Trigger  "and"

== system new_control/RIGHT LEG/MOTOR POSITION REFERENCE GENERATOR ==
  note: KALMAN FILTER
  GAIT PHASE : Inport
  LAG COMPENSATION : Inport  Port=2
  AMPLITUDE : Inport  Port=3
  Gain : Gain  Gain=-1
  Motion mapping2 : Lookup_n-D  NumberOfTableDimensions=1  BreakpointsForDimension1=[-1, -0.8, -0.6, -0.4, -0.2, -0.1, 0, 0.1, 0.2, 0.4, 0.6, 0.8, 1]  BreakpointsForDimension2=qbreak(:,2)  Table=[-1, -0.8, -0.6, -0.4, -0.2, -0.1, 0, 0, 0.005, 0.01, 0.015,0.02,0.025]  InterpMethod=Cubic spline  ExtrapMethod=Cubic spline  InternalRulePriority=Speed  RndMeth=Simplest
  Plus : Sum
  Product : Product
  Rate Transition : RateTransition  OutPortSampleTime=0.01
  Ref traj w/ noise : ctrlSharedLib/Kalman Filter  Commented=on  TimeDomain=Discrete-Time  UseCurrentEstimator=off  ModelSource=Individual A, B, C, D matrices  ModelSourceVariable=ss(0.95,1,1,0,1)  A=[1]  B=1  C=[1]  D=0  NumberOfStates=1  NumberOfInputs=1  NumberOfOutputs=1  InitialEstimateSource=Dialog  X0=[0]  P0=10  UseK=off  UseGH=off  NumberOfProcessNoiseInputs=1  G=1  TimeInvariantG=on  H=0  TimeInvariantH=on  Q=1e-3  TimeInvariantQ=on  R=9e-4  TimeInvariantR=on  N=0  TimeInvariantN=on  AddInputPort=off  AddEnablePort=off  OutputEstimatedY=off  OutputP=off  Ts=-1
  Saturation : Saturate  UpperLimit=600*pi/180  LowerLimit=-600*pi/180
  Sin1 : Trigonometry
  Ref motion : Outport
  wires:
  Motion mapping2/1 -> Product/1
  Product/1 -> Saturation/1
  Sin1/1 -> Gain/1
  Plus/1 -> Sin1/1
  GAIT PHASE/1 -> Plus/1
  LAG COMPENSATION/1 -> Plus/2
  AMPLITUDE/1 -> Product/2
  Gain/1 -> Rate Transition/1
  Saturation/1 -> Ref motion/1
  Rate Transition/1 -> Motion mapping2/1

== system new_control/RIGHT LEG/Subsystem ==
  Angle estimation : Inport
  Velocity surrogate (quarature component) : Inport  Port=2
  Ref amplitude : Inport  Port=3
  classif : Inport  Port=4
  Sig_Power : Inport  Port=5
  Cast To Double : DataTypeConversion  OutDataTypeStr=double  SaturateOnIntegerOverflow=off  RndMeth=Floor
  Chart1 : Stateflow chart  TreatAsAtomicUnit=on
  Constant : Constant
  Product : Product
  Product1 : Product
  SIGMOID SCALING : Subsystem
  Sqrt : Sqrt
  Square : Math  Operator=square
  Square1 : Math  Operator=square
  Sum : Sum
  Amplitude_R : Outport
  wires:
  Square/1 -> Sum/1
  Square1/1 -> Sum/2
  Sum/1 -> Sqrt/1
  Product/1 -> Amplitude_R/1
  SIGMOID SCALING/1(Out1) -> Product/1  "Sig_Scale_R"
  Cast To Double/1 -> Chart1/1(class)
  classif/1 -> Cast To Double/1
  Ref amplitude/1 -> Chart1/2(amplitude)
  Chart1/3(sigmoid_power) -> SIGMOID SCALING/2(sigmoid_power)
  Sqrt/1 -> Product1/1  "PORTRAIT RADIUS R"
  Chart1/2(gain) -> Product/2
  Velocity surrogate (quarature component)/1 -> Square1/1
  Sig_Power/1 -> Chart1/3(sig_power)
  Angle estimation/1 -> Square/1
  Product1/1 -> SIGMOID SCALING/1(PORTRAIT RADIUS)
  Constant/1 -> Chart1/4("scale_LM ")
  Chart1/1(scale_LM) -> Product1/2

== system new_control/Subsystem1/Left Motor Velocity1 ==
  SWITCH : Inport
  Motor command : Inport  Port=2
  Motor Actual Position Receive : Subsystem  Priority=2
  Subsystem : Subsystem  Priority=1
  MOTOR POSITION : Outport
  MOTOR SPEED : Outport  Port=2
  MOTOR TORQUE : Outport  Port=3
  wires:
  Motor command/1 -> Subsystem/1(Motor command)
  SWITCH/1 -> Motor Actual Position Receive/1(SWITCH), Subsystem/2(SWITCH)
  Motor Actual Position Receive/1(MOTOR POSITION) -> MOTOR POSITION/1
  Motor Actual Position Receive/2(MOTOR SPEED) -> MOTOR SPEED/1
  Motor Actual Position Receive/3(MOTOR TORQUE) -> MOTOR TORQUE/1

== system new_control/Subsystem1/PID1 ==
  Ref : Inport
  Actual Motion : Inport  Port=2
  Enable : EnablePort  StatesWhenEnabling=reset
  Gain4 : Gain  Gain=14
  Gain7 : Gain  Gain=0.02
  Gain8 : Gain  Gain=0
  Integrator1 : Integrator
  Subsystem2 : Subsystem  mask{wn=20, zt=1, x0=0}
      mask prompts: wn "Cut-off frequency (rad/s)"; zt "Damping ratio"; x0 "Initial Condition"
  Sum : Sum  Inputs=|-+  OutDataTypeStr=double
  Sum5 : Sum  Inputs=|+|+|-
  Terminator2 : Terminator
  Velocity output : Outport
  wires:
  Gain7/1 -> Sum5/3
  Subsystem2/2(yd) -> Gain7/1
  Integrator1/1 -> Gain8/1
  Gain4/1 -> Sum5/1
  Actual Motion/1 -> Sum/1
  Gain8/1 -> Sum5/2
  Subsystem2/1(y) -> Terminator2/1
  Sum/1 -> Integrator1/1, Gain4/1
  Ref/1 -> Sum/2
  Sum5/1 -> Velocity output/1, Subsystem2/1(x)

== system new_control/Subsystem1/PID2 ==
  Ref : Inport
  Actual Motion : Inport  Port=2
  Enable : EnablePort  StatesWhenEnabling=reset
  Gain4 : Gain  Gain=14
  Gain7 : Gain  Gain=0.02
  Gain8 : Gain  Gain=0
  Integrator1 : Integrator
  Subsystem2 : Subsystem  mask{wn=20, zt=1, x0=0}
      mask prompts: wn "Cut-off frequency (rad/s)"; zt "Damping ratio"; x0 "Initial Condition"
  Sum : Sum  Inputs=|-+  OutDataTypeStr=double
  Sum5 : Sum  Inputs=|+|+|-
  Terminator2 : Terminator
  Velocity output : Outport
  wires:
  Gain7/1 -> Sum5/3
  Subsystem2/2(yd) -> Gain7/1
  Integrator1/1 -> Gain8/1
  Gain4/1 -> Sum5/1
  Actual Motion/1 -> Sum/1
  Gain8/1 -> Sum5/2
  Subsystem2/1(y) -> Terminator2/1
  Sum/1 -> Integrator1/1, Gain4/1
  Ref/1 -> Sum/2
  Sum5/1 -> Velocity output/1, Subsystem2/1(x)

== system new_control/Subsystem1/Right Motor Velocity1 ==
  SWITCH : Inport
  Motor command : Inport  Port=2
  Motor Actual Position Receive : Subsystem  Priority=4
  Subsystem : Subsystem  Priority=3
  MOTOR POSITION : Outport
  MOTOR SPEED : Outport  Port=2
  MOTOR TORQUE : Outport  Port=3
  wires:
  Motor command/1 -> Subsystem/1(Motor command)
  SWITCH/1 -> Motor Actual Position Receive/1(SWITCH), Subsystem/2(SWITCH)
  Motor Actual Position Receive/1(MOTOR POSITION) -> MOTOR POSITION/1
  Motor Actual Position Receive/2(MOTOR SPEED) -> MOTOR SPEED/1
  Motor Actual Position Receive/3(MOTOR TORQUE) -> MOTOR TORQUE/1

== system new_control/Subsystem3/Left Motor Velocity ==
  SWITCH : Inport
  Motor command : Inport  Port=2
  Motor Actual Position Receive : Subsystem  Priority=4
  Subsystem : Subsystem  Priority=3
  MOTOR POSITION : Outport
  MOTOR SPEED : Outport  Port=2
  MOTOR TORQUE : Outport  Port=3
  wires:
  Motor command/1 -> Subsystem/1(Motor command)
  SWITCH/1 -> Motor Actual Position Receive/1(SWITCH), Subsystem/2(SWITCH)
  Motor Actual Position Receive/1(MOTOR POSITION) -> MOTOR POSITION/1
  Motor Actual Position Receive/2(MOTOR SPEED) -> MOTOR SPEED/1
  Motor Actual Position Receive/3(MOTOR TORQUE) -> MOTOR TORQUE/1

== system new_control/Subsystem3/Right Motor Velocity ==
  SWITCH : Inport
  Motor command : Inport  Port=2
  Motor Actual Position Receive : Subsystem  Priority=2
  Subsystem : Subsystem  Priority=1
  MOTOR POSITION : Outport
  MOTOR SPEED : Outport  Port=2
  MOTOR TORQUE : Outport  Port=3
  wires:
  Motor command/1 -> Subsystem/1(Motor command)
  SWITCH/1 -> Motor Actual Position Receive/1(SWITCH), Subsystem/2(SWITCH)
  Motor Actual Position Receive/1(MOTOR POSITION) -> MOTOR POSITION/1
  Motor Actual Position Receive/2(MOTOR SPEED) -> MOTOR SPEED/1
  Motor Actual Position Receive/3(MOTOR TORQUE) -> MOTOR TORQUE/1

== system new_control/Subsystem3/Subsystem1 ==
  x : Inport
  Constant : Constant  Value=2
  Integrator1 : Integrator  InitialConditionSource=external
  Integrator2 : Integrator
  Product : Product  RndMeth=Zero
  Product1 : Product  RndMeth=Zero
  Product2 : Product  Inputs=3  RndMeth=Zero
  Sum : Sum  Inputs=|+-
  Sum1 : Sum  Inputs=|+-
  wn : Constant  Value=wn
  x0 : Constant  Value=x0
  zt : Constant  Value=zt
  y : Outport  VectorParamsAs1DForOutWhenUnconnected=off
  yd : Outport  Port=2  VectorParamsAs1DForOutWhenUnconnected=off
  wires:
  Sum/1 -> Product/2
  wn/1 -> Product/1, Product1/1
  Sum1/1 -> Sum/1
  x0/1 -> Integrator1/2
  Integrator2/1 -> Product1/2, Product2/1
  Product/1 -> Integrator2/1
  x/1 -> Sum1/1
  Product1/1 -> Integrator1/1, yd/1
  Integrator1/1 -> Sum1/2, y/1
  Product2/1 -> Sum/2
  zt/1 -> Product2/3
  Constant/1 -> Product2/2

== system new_control/Subsystem3/Subsystem4 ==
  x : Inport
  Constant : Constant  Value=2
  Integrator1 : Integrator  InitialConditionSource=external
  Integrator2 : Integrator
  Product : Product  RndMeth=Zero
  Product1 : Product  RndMeth=Zero
  Product2 : Product  Inputs=3  RndMeth=Zero
  Sum : Sum  Inputs=|+-
  Sum1 : Sum  Inputs=|+-
  wn : Constant  Value=wn
  x0 : Constant  Value=x0
  zt : Constant  Value=zt
  y : Outport  VectorParamsAs1DForOutWhenUnconnected=off
  yd : Outport  Port=2  VectorParamsAs1DForOutWhenUnconnected=off
  wires:
  Sum/1 -> Product/2
  wn/1 -> Product/1, Product1/1
  Sum1/1 -> Sum/1
  x0/1 -> Integrator1/2
  Integrator2/1 -> Product1/2, Product2/1
  Product/1 -> Integrator2/1
  x/1 -> Sum1/1
  Product1/1 -> Integrator1/1, yd/1
  Integrator1/1 -> Sum1/2, y/1
  Product2/1 -> Sum/2
  zt/1 -> Product2/3
  Constant/1 -> Product2/2

== system new_control/IMUs/SOGI + FLL (IN PHASE + QUADRATURE COMPONENT ESTIMATION)/REMOVE DRIFT ==
  x : Inport
  Constant : Constant  Value=2
  Integrator1 : Integrator  InitialConditionSource=external
  Integrator2 : Integrator
  Product : Product  RndMeth=Zero
  Product1 : Product  RndMeth=Zero
  Product2 : Product  Inputs=3  RndMeth=Zero
  Sum : Sum  Inputs=|+-
  Sum1 : Sum  Inputs=|+-
  wn : Constant  Value=wn
  x0 : Constant  Value=x0
  zt : Constant  Value=zt
  y : Outport  VectorParamsAs1DForOutWhenUnconnected=off
  wires:
  Sum/1 -> Product/2
  wn/1 -> Product/1, Product1/1
  Sum1/1 -> Sum/1
  x0/1 -> Integrator1/2
  Integrator2/1 -> Product1/2, Product2/1
  Product/1 -> Integrator2/1
  x/1 -> Sum1/1
  Product1/1 -> Integrator1/1
  Integrator1/1 -> Sum1/2, y/1
  Product2/1 -> Sum/2
  zt/1 -> Product2/3
  Constant/1 -> Product2/2

== system new_control/IMUs/SOGI + FLL (IN PHASE + QUADRATURE COMPONENT ESTIMATION)1/REMOVE DRIFT ==
  x : Inport
  Constant : Constant  Value=2
  Integrator1 : Integrator  InitialConditionSource=external
  Integrator2 : Integrator
  Product : Product  RndMeth=Zero
  Product1 : Product  RndMeth=Zero
  Product2 : Product  Inputs=3  RndMeth=Zero
  Sum : Sum  Inputs=|+-
  Sum1 : Sum  Inputs=|+-
  wn : Constant  Value=wn
  x0 : Constant  Value=x0
  zt : Constant  Value=zt
  y : Outport  VectorParamsAs1DForOutWhenUnconnected=off
  wires:
  Sum/1 -> Product/2
  wn/1 -> Product/1, Product1/1
  Sum1/1 -> Sum/1
  x0/1 -> Integrator1/2
  Integrator2/1 -> Product1/2, Product2/1
  Product/1 -> Integrator2/1
  x/1 -> Sum1/1
  Product1/1 -> Integrator1/1
  Integrator1/1 -> Sum1/2, y/1
  Product2/1 -> Sum/2
  zt/1 -> Product2/3
  Constant/1 -> Product2/2

== system new_control/Initialize Function/Config_L /Enter Config Mode ==
  Compare To Zero8 : simulink/Logic and Bit Operations/Compare To Zero  relop===  OutDataTypeStr=boolean
  Constant5 : Constant  Value=0x00
  Start_Config_L : arduinolib/I2C Write  I2CModule=0  Mode=Master  SlaveAddress=0x28  SlaveByteOrder=BigEndian  Direction=Transmitter  RegisterAddressMode=on  RegisterAddress=0x3D  SlaveDataType=uint8  DataLength=1  NoAck=off  RepeatedStart=off  OutputStatus=on  blockPlatform=ARDUINO
  Status : Outport
  wires:
  Start_Config_L/1 -> Compare To Zero8/1  "0 for success"
  Constant5/1 -> Start_Config_L/1
  Compare To Zero8/1 -> Status/1

== system new_control/Initialize Function/Config_L /Start Fused (NDOF) Mode ==
  Enable : EnablePort
  Compare To Constant2 : simulink/Logic and Bit Operations/Compare To Constant  relop===  const=0  OutDataTypeStr=boolean
  Constant4 : Constant  Value=0x0C
  I2C Write8 : arduinolib/I2C Write  I2CModule=0  Mode=Master  SlaveAddress=0x28  SlaveByteOrder=BigEndian  Direction=Transmitter  RegisterAddressMode=on  RegisterAddress=0x3D  SlaveDataType=uint8  DataLength=1  NoAck=off  RepeatedStart=off  OutputStatus=on  blockPlatform=ARDUINO
  Status : Outport
  wires:
  Compare To Constant2/1 -> Status/1
  Constant4/1 -> I2C Write8/1
  I2C Write8/1 -> Compare To Constant2/1  "0: success"

== system new_control/Initialize Function/Config_L /X=Z, Y=Y, Z=X ==
  Enable : EnablePort
  Compare To Constant : simulink/Logic and Bit Operations/Compare To Constant  relop=~=  const=hex2dec('06')  OutDataTypeStr=boolean
  Compare To Constant1 : simulink/Logic and Bit Operations/Compare To Constant  relop===  const=hex2dec('06')  OutDataTypeStr=boolean
  Enabled Subsystem : Subsystem  TreatAsAtomicUnit=on
  I2C Read : arduinolib/I2C Read  I2CModule=0  Mode=Master  SlaveAddress=0x28  SlaveByteOrder=LittleEndian  Direction=Receiver  RegisterAddressMode=on  RegisterAddress=0x41  SlaveDataType=uint8  DataLength=1  NoAck=off  RepeatedStart=off  OutputStatus=off  blockPlatform=ARDUINO  SampleTime=-1
  OR : Logic  Operator=OR  IconShape=distinctive  AllPortsSameDT=off  OutDataTypeStr=boolean
  Status : Outport
  wires:
  I2C Read/1 -> Compare To Constant1/1, Compare To Constant/1
  Compare To Constant1/1 -> OR/2
  Compare To Constant/1 -> Enabled Subsystem/Enable
  Enabled Subsystem/1(Status) -> OR/1
  OR/1 -> Status/1

== system new_control/Initialize Function/Config_L /Z = -Z ==
  note: 0x01: Z = -Z
  Enable : EnablePort
  Compare To Constant : simulink/Logic and Bit Operations/Compare To Constant  relop=~=  const=hex2dec('01')  OutDataTypeStr=boolean
  Compare To Constant1 : simulink/Logic and Bit Operations/Compare To Constant  relop===  const=hex2dec('01')  OutDataTypeStr=boolean
  OR : Logic  Operator=OR  IconShape=distinctive  AllPortsSameDT=off  OutDataTypeStr=boolean
  Read : arduinolib/I2C Read  I2CModule=0  Mode=Master  SlaveAddress=0x28  SlaveByteOrder=LittleEndian  Direction=Receiver  RegisterAddressMode=on  RegisterAddress=0x42  SlaveDataType=uint8  DataLength=1  NoAck=off  RepeatedStart=off  OutputStatus=off  blockPlatform=ARDUINO  SampleTime=-1
  Write : Subsystem  TreatAsAtomicUnit=on
  Status : Outport
  wires:
  Write/1(Status) -> OR/1
  Compare To Constant/1 -> Write/Enable
  Read/1 -> Compare To Constant1/1, Compare To Constant/1
  Compare To Constant1/1 -> OR/2
  OR/1 -> Status/1
